simulink model "untitled"  (R2017b)
settings: Solver=VariableStepAuto  StartTime=0.0  StopTime=10.0  RelTol=1e-3
values from neighbouring files (symbols this model uses):
  z0 = -200    [trim_untitled.m]
libraries: shared3dof x1
settings Model: Creator=ken  LastModifiedBy=ken

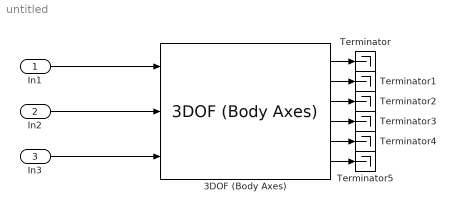
== system untitled ==
  In1 : Inport
  In2 : Inport  Port=2
  In3 : Inport  Port=3
  3DOF (Body Axes) : shared3dof/3DOF (Body Axes)  units=Metric (MKS)  mtype=Fixed  v_ini=vair0  theta_ini=pitchTheta0  alpha_ini=0  q_ini=0  pos_ini=[0 z0]  mass=1.0  mass_e=0.5  mass_f=3.0  Iyy=1.0  Iyy_e=0.5  Iyy_f=3.0  g_in=Internal  g=11  vre_flag=on  abi_flag=off
      settings: SourceProductName=Aerospace Blockset  SourceProductBaseCode=AE
  Terminator{,1..5} (6 alike) : Terminator
  wires:
  In1/1 -> 3DOF (Body Axes)/1
  In2/1 -> 3DOF (Body Axes)/2
  In3/1 -> 3DOF (Body Axes)/3
  3DOF (Body Axes)/1 -> Terminator/1
  3DOF (Body Axes)/2 -> Terminator1/1
  3DOF (Body Axes)/3 -> Terminator2/1
  3DOF (Body Axes)/4 -> Terminator3/1
  3DOF (Body Axes)/5 -> Terminator4/1
  3DOF (Body Axes)/6 -> Terminator5/1
